simulink model "dynamiczny_dyskretny_zlinearyzowany"  (R2017b)
settings: Solver=VariableStepAuto  StartTime=0.0  StopTime=time  RelTol=1e-3
values from neighbouring files (symbols this model uses):
  alfa1 = -0.9    [params.m]
  alfa2 = 1.37    [params.m]
  alfa3 = -1.95    [params.m]
  alfa4 = 0.05    [params.m]
  DelayValue = 1    [params.m]
  K = 5    [params.m]
  StartDelay = 5    [params.m]
  StartValue = 0    [params.m]
  T = 1    [params.m]
  T1 = 10    [params.m]
  T2 = 6    [params.m]
  ulin = 0    [params.m]
settings Model: Creator=Tomek  LastModifiedBy=Tomek

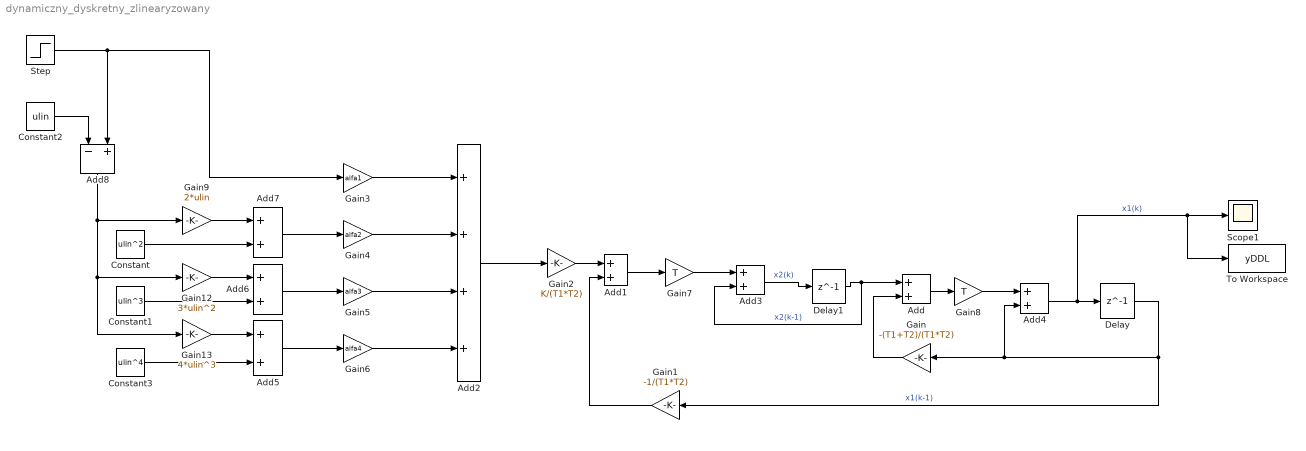
== system dynamiczny_dyskretny_zlinearyzowany ==
  Add{,1,3..7} (7 alike) : Sum
  Add2 : Sum  Inputs=++++
  Add8 : Sum  Inputs=-+
  Constant : Constant  Value=ulin^2
  Constant1 : Constant  Value=ulin^3
  Constant2 : Constant  Value=ulin
  Constant3 : Constant  Value=ulin^4
  Delay : Delay  DelayLength=1  SampleTime=T
  Delay1 : Delay  DelayLength=1  SampleTime=T
  Gain : Gain  Gain=-(T1+T2)/(T1*T2)
  Gain1 : Gain  Gain=-1/(T1*T2)
  Gain12 : Gain  Gain=3*ulin^2
  Gain13 : Gain  Gain=4*ulin^3
  Gain2 : Gain  Gain=K/(T1*T2)
  Gain3 : Gain  Gain=alfa1
  Gain4 : Gain  Gain=alfa2
  Gain5 : Gain  Gain=alfa3
  Gain6 : Gain  Gain=alfa4
  Gain7 : Gain  Gain=T
  Gain8 : Gain  Gain=T
  Gain9 : Gain  Gain=2*ulin
  Scope1 : Scope
  Step : Step  Time=StartDelay  Before=StartValue  After=DelayValue  SampleTime=0
  To Workspace : ToWorkspace  VariableName=yDDL  SaveFormat=Timeseries  SampleTime=-1
  wires:
  Add1/1 -> Gain7/1
  Add4/1 -> To Workspace/1, Scope1/1, Delay/1  "x1(k)"
  Gain7/1 -> Add3/1
  Gain5/1 -> Add2/3
  Gain3/1 -> Add2/1
  Gain/1 -> Add/2
  Delay1/1 -> Add3/2, Add/1  "x2(k-1)"
  Gain2/1 -> Add1/1
  Gain6/1 -> Add2/4
  Add2/1 -> Gain2/1
  Gain4/1 -> Add2/2
  Delay/1 -> Gain1/1, Add4/2, Gain/1  "x1(k-1)"
  Gain1/1 -> Add1/2
  Add3/1 -> Delay1/1  "x2(k)"
  Add/1 -> Gain8/1
  Gain8/1 -> Add4/1
  Step/1 -> Gain3/1, Add8/2
  Constant2/1 -> Add8/1
  Add6/1 -> Gain5/1
  Add7/1 -> Gain4/1
  Add5/1 -> Gain6/1
  Constant3/1 -> Add5/2
  Constant1/1 -> Add6/2
  Constant/1 -> Add7/2
  Gain12/1 -> Add6/1
  Gain13/1 -> Add5/1
  Gain9/1 -> Add7/1
  Add8/1 -> Gain9/1, Gain12/1, Gain13/1
